simulink model "LastNull"  (R2015a)
settings: configuration reference "SIMULATION_CONFIGURATION" (kept outside this file)
settings Model: CovSFcnEnable=off  Creator=moritz  LastModifiedBy=moritz
settings ConfigSetRef: SourceLocation=Base Workspace

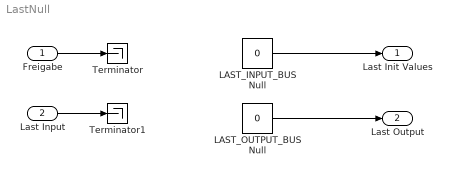
== system LastNull ==
  Freigabe : Inport  OutDataTypeStr=boolean
  Last Input : Inport  Port=2  OutDataTypeStr=Bus: LAST_INPUT_BUS  BusOutputAsStruct=on
  LAST_INPUT_BUS Null : Constant  Value=0  OutDataTypeStr=Bus: LAST_INPUT_BUS  SampleTime=-1
  LAST_OUTPUT_BUS Null : Constant  Value=0  OutDataTypeStr=Bus: LAST_OUTPUT_BUS  SampleTime=-1
  Terminator : Terminator
  Terminator1 : Terminator
  Last Init Values : Outport  OutDataTypeStr=Bus: LAST_INPUT_BUS  BusOutputAsStruct=on
  Last Output : Outport  Port=2  OutDataTypeStr=Bus: LAST_OUTPUT_BUS  BusOutputAsStruct=on
  wires:
  LAST_INPUT_BUS Null/1 -> Last Init Values/1
  Freigabe/1 -> Terminator/1
  Last Input/1 -> Terminator1/1
  LAST_OUTPUT_BUS Null/1 -> Last Output/1
